simulink model "Model_for_PIL"  (R2019a)
settings: Solver=FixedStepDiscrete  StartTime=0.0  StopTime=10.0  RelTol=1e-3  EnableMultiTasking=on
undefined symbols (not defined in the file): Ts
settings Model: SimulationMode=processor-in-the-loop (pil)  ExtModeTrigDuration=10  Creator=user  LastModifiedBy=djtn
settings OptimizationCC: DefaultParameterBehavior=Inlined  UseDivisionForNetSlopeComputation=on  EnhancedBackFolding=on  PassReuseOutputArgsAs=Individual arguments  MaxStackSize=64  OptimizeBlockOrder=speed  DifferentSizesBufferReuse=on  OptimizationCustomize=off
settings DebuggingCC: SignalInfNanChecking=error  IntegerOverflowMsg=error  ParameterTunabilityLossMsg=error  AssertControl=DisableAll  SFUndirectedBroadcastEventsDiag=error
settings HardwareCC: ProdBitPerPointer=32  ProdBitPerSizeT=32  ProdBitPerPtrDiffT=32  ProdLargestAtomicInteger=Long  ProdWordSize=32  ProdHWDeviceType=STM32CortexM
settings SFSimCC: CompileTimeRecursionLimit=0  EnableRuntimeRecursion=off  MATLABDynamicMemAlloc=off
settings RTWCC: SystemTargetFile=stm32.tlc  TemplateMakefile=stm32.tmf  Description=stm32 (Embedded Target)  GenerateReport=on  Toolchain=GNU Tools for ARM Embedded Processors  IncludeHyperlinkInReport=on  CreateSILPILBlock=PIL  GenerateTraceInfo=on  GenerateTraceReport=on  GenerateTraceReportSl=on  GenerateTraceReportSf=on  GenerateTraceReportEml=on  CheckMdlBeforeBuild=Warning
settings CodeAppCC: ForceParamTrailComments=on  IgnoreCustomStorageClasses=off  MaxIdLength=64  OperatorAnnotations=on  SimulinkDataObjDesc=on  SFDataObjDesc=on  CustomSymbolStrType=$N$R$M  SimulinkBlockComments=off
settings STFCustomTargetCC: CodeReplacementLibrary=ARM CMSIS SIN COS  MultiwordLength=256  ParMdlRefBuildCompliant=on  IncludeMdlTerminateFcn=off  CombineOutputUpdateFcns=on  ERTCustomFileBanners=on  SupportContinuousTime=off  SupportNonInlinedSFcns=off  RemoveResetFunc=on  MATLABClassNameForMDSCustomization=Simulink.SoftwareTarget.ERTCustomization  GRTInterface=off  SystemTargetFile=stm32.tlc
settings ERTTargetCC: CodeReplacementLibrary=ARM CMSIS SIN COS  CompOptLevelCompliant=off  ConcurrentExecutionCompliant=off  IncludeMdlTerminateFcn=off  ModelStepFunctionPrototypeControlCompliant=off  CPPClassGenCompliant=off  UseToolchainInfoCompliant=off  ExtModeStaticAllocSize=256  ExtModeMexFile=ext_serial_win32_comm  ExtModeMexArgs=0,1,115200,10  InlinedParameterPlacement=NonHierarchical  ERTSrcFileBannerTemplate=sourceFileTemplate.cgt  ERTHdrFileBannerTemplate=sourceFileTemplate.cgt  ERTDataSrcFileTemplate=sourceFileTemplate.cgt  ERTDataHdrFileTemplate=sourceFileTemplate.cgt  ERTCustomFileTemplate=customRoutineProcess.tlc

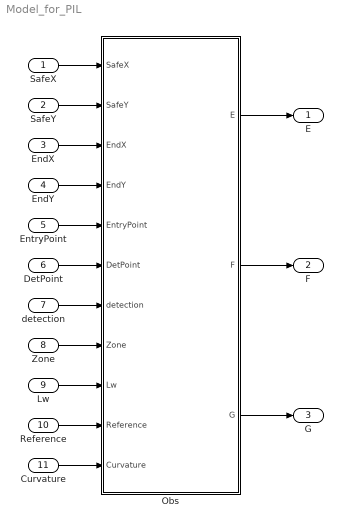
== system Model_for_PIL ==
  SafeX : Inport
  SafeY : Inport  Port=2
  EndX : Inport  Port=3
  EndY : Inport  Port=4
  EntryPoint : Inport  Port=5
  DetPoint : Inport  Port=6
  detection : Inport  Port=7
  Zone : Inport  Port=8
  Lw : Inport  Port=9
  Reference : Inport  Port=10
  Curvature : Inport  Port=11
  Obs : Subsystem  TreatAsAtomicUnit=on
  E : Outport  PortDimensions=[2,2]
  F : Outport  Port=2  PortDimensions=[2,4]
  G : Outport  Port=3  PortDimensions=[2,1]
  wires:
  SafeX/1 -> Obs/1(SafeX)
  SafeY/1 -> Obs/2(SafeY)
  EndX/1 -> Obs/3(EndX)
  EndY/1 -> Obs/4(EndY)
  EntryPoint/1 -> Obs/5(EntryPoint)
  DetPoint/1 -> Obs/6(DetPoint)
  detection/1 -> Obs/7(detection)
  Zone/1 -> Obs/8(Zone)
  Lw/1 -> Obs/9("Lw ")
  Reference/1 -> Obs/10(Reference)
  Curvature/1 -> Obs/11(Curvature)
  Obs/1(E) -> E/1
  Obs/2(F) -> F/1
  Obs/3(G) -> G/1

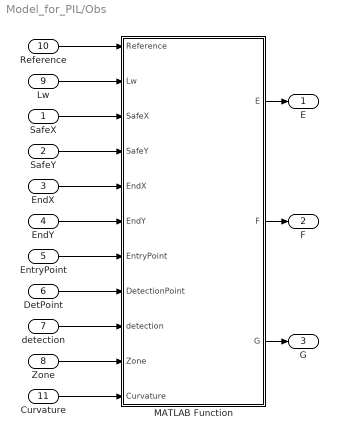
== system Model_for_PIL/Obs ==
  SafeX : Inport  PortDimensions=1  SampleTime=Ts
  SafeY : Inport  Port=2  PortDimensions=1  SampleTime=Ts
  EndX : Inport  Port=3  PortDimensions=1  SampleTime=Ts
  EndY : Inport  Port=4  PortDimensions=1  SampleTime=Ts
  EntryPoint : Inport  Port=5  PortDimensions=[1,4]  SampleTime=Ts
  DetPoint : Inport  Port=6  PortDimensions=[1,4]  SampleTime=Ts
  detection : Inport  Port=7  PortDimensions=1  SampleTime=Ts
  Zone : Inport  Port=8  PortDimensions=1  SampleTime=Ts
  "Lw " : Inport  Port=9  PortDimensions=1  SampleTime=Ts
  Reference : Inport  Port=10  PortDimensions=[1,4]  SampleTime=Ts
  Curvature : Inport  Port=11  PortDimensions=1  SampleTime=Ts
  MATLAB Function : MATLAB Function  TreatAsAtomicUnit=on
  E : Outport  PortDimensions=[2,2]  SampleTime=Ts
  F : Outport  Port=2  PortDimensions=[2,4]  SampleTime=Ts
  G : Outport  Port=3  PortDimensions=[2,1]  SampleTime=Ts
  wires:
  EndX/1 -> MATLAB Function/5(EndX)
  detection/1 -> MATLAB Function/9(detection)
  EndY/1 -> MATLAB Function/6(EndY)
  SafeY/1 -> MATLAB Function/4(SafeY)
  DetPoint/1 -> MATLAB Function/8(DetectionPoint)
  Zone/1 -> MATLAB Function/10(Zone)
  SafeX/1 -> MATLAB Function/3(SafeX)
  "Lw "/1 -> MATLAB Function/2(Lw)
  Reference/1 -> MATLAB Function/1(Reference)
  EntryPoint/1 -> MATLAB Function/7(EntryPoint)
  Curvature/1 -> MATLAB Function/11(Curvature)
  MATLAB Function/3(G) -> G/1
  MATLAB Function/2(F) -> F/1
  MATLAB Function/1(E) -> E/1

== matlab function Model_for_PIL/Obs/MATLAB Function ==
  settings: updateMethod=DISCRETE  sampleTime=Ts
  data: Reference input; E output size=[2 2]; Lw input; SafeX input; SafeY input; EndX input; EndY input; EntryPoint input; DetectionPoint input; detection input; F output size=[2 4]; G output size=[2 1]; Zone input; Curvature input
function [E, F, G] = fcn(Reference,Lw,SafeX,SafeY,EndX,EndY,EntryPoint,DetectionPoint,detection,Zone,Curvature)

[E, F, G] = LaneKeepConstraint(Reference,Lw,detection,SafeX,SafeY,EndX,EndY,EntryPoint,Zone,DetectionPoint,Curvature);
